simulink model "KF"  (R2025b)
settings: Solver=VariableStepAuto  StartTime=0.0  StopTime=35  RelTol=1e-3
StopFcn:
  | % -----------------------------
  | %   Kalman Filter Visualization
  | % -----------------------------
  | 
  | % 안전하게 데이터 존재 여부 확인
  | if evalin('base','exist(''out'',''var'')')
  | 
  |     % out 구조체 불러오기
  |     data = evalin('base','out');
  | 
  |     % Timeseries 는 .Time, .Data 로 접근
  |     t = data.z_out.Time;
  | 
  |     % 관측 z_k = [x, y]
  |     z_x = data.z_out.Data(:,1);
  |     z_y = data.z_out.Data(:,2);
  | 
  |     % x_pred = [x vx y vy]
  |     xpred_x = data.x_pred.Data(:,1);
  |     xpred_y = data.x_pred.Data(:,3);
  | 
  |     % x_est = [x vx y vy]
  |     xest_x = data.x_est.Data(:,1);
  |     xest_y = data.x_est.Data(:,3);
  | 
  |     figure; hold on; grid on;
  | 
  |     % ---- X plot ----
  |     subplot(2,1,1); hold on; grid on;
  |     plot(t, z_x,'ro','DisplayName','Observed X');
  |     plot(t, xpred_x,'b--','LineWidth',1.3,'DisplayName','Predicted X');
  |     plot(t, xest_x,'g-','LineWidth',1.3,'DisplayName','Estimated X');
  |     xlabel('Time'); ylabel('X'); title('X Position');
  |     legend;
  | 
  |     % ---- Y plot ----
  |     subplot(2,1,2); hold on; grid on;
  |     plot(t, z_y,'ro','DisplayName','Observed Y');
  |     plot(t, xpred_y,'b--','LineWidth',1.3,'DisplayName','Predicted Y');
  |     plot(t, xest_y,'g-','LineWidth',1.3,'DisplayName','Estimated Y');
  |     xlabel('Time'); ylabel('Y'); title('Y Position');
  |     legend;
  | 
  | else
  |     disp('ERROR: out 구조체가 workspace에 없습니다.');
  | end
libraries: simulink x2, matrix_library x2
settings Model: Creator=xox  LastModifiedBy=xox
settings OptimizationCC: BlockReduction=off  DefaultParameterBehavior=Inlined  BufferReuse=off

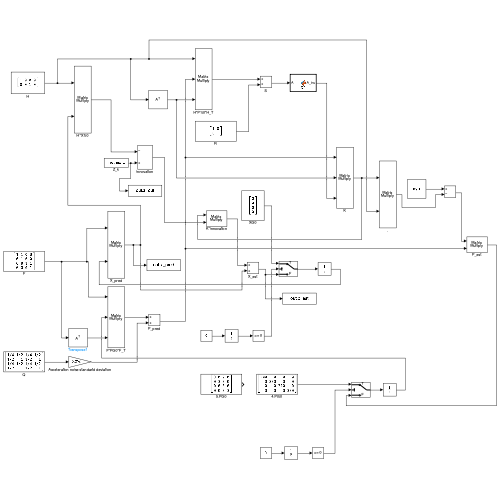
[thumbnail: Simulink's stored preview of the top-level diagram]
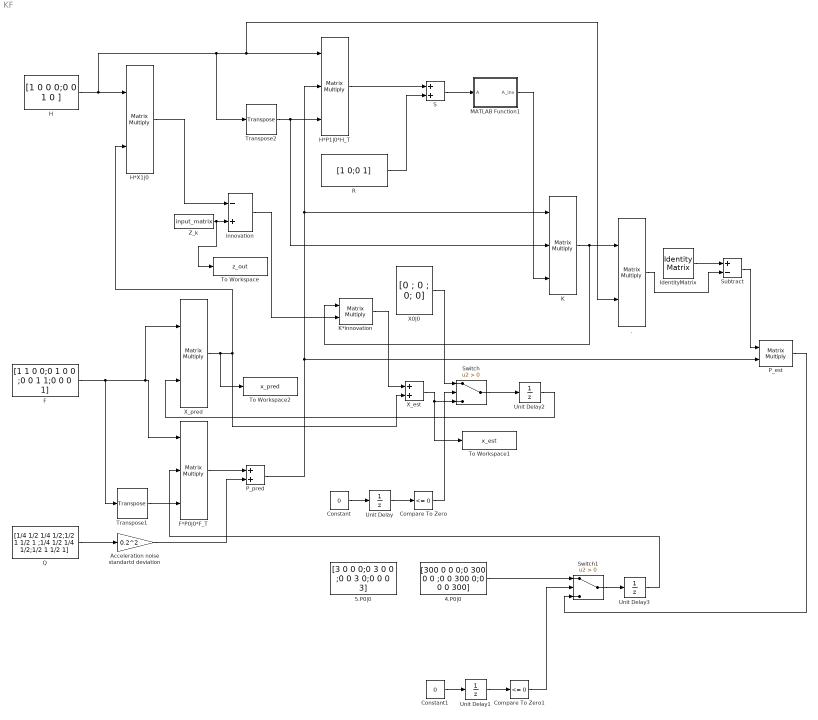
== system KF ==
  . : Product  Multiplication=Matrix(*)
  4.P0|0 : Constant  Value=[300 0 0 0;0 300 0 0 ;0 0 300 0;0 0 0 300]  VectorParams1D=off
  5.P0|0 : Constant  Value=[3 0 0 0;0 3 0 0 ;0 0 3 0;0 0 0 3]  VectorParams1D=off
  Acceleration noise standartd deviation : Gain  Gain=0.2^2
  Compare To Zero : simulink/Logic and Bit Operations/Compare To Zero  relop=<=  OutDataTypeStr=boolean
  Compare To Zero1 : simulink/Logic and Bit Operations/Compare To Zero  relop=<=  OutDataTypeStr=boolean
  Constant : Constant  Value=0
  Constant1 : Constant  Value=0
  F : Constant  Value=[1 1 0 0;0 1 0 0 ;0 0 1 1;0 0 0 1]  VectorParams1D=off
  F*P0|0*F_T : Product  Inputs=3  Multiplication=Matrix(*)
  H : Constant  Value=[1 0 0 0;0 0 1 0 ]  VectorParams1D=off
  H*P1|0*H_T : Product  Inputs=3  Multiplication=Matrix(*)
  H*X1|0 : Product  Multiplication=Matrix(*)
  IdentityMatrix : IdentityMatrix  OutputDimensions=4
  K : Product  Inputs=3  Multiplication=Matrix(*)
  K*innovation : Product  Multiplication=Matrix(*)
  MATLAB Function1 : MATLAB Function  TreatAsAtomicUnit=on
  P_est : Product  Multiplication=Matrix(*)
  P_pred : Sum
  Q : Constant  Value=[1/4 1/2 1/4 1/2;1/2 1 1/2 1 ;1/4 1/2 1/4 1/2;1/2 1 1/2 1]  VectorParams1D=off
  R : Constant  Value=[1 0;0 1]  VectorParams1D=off
  S : Sum
  Subtract : Sum  Inputs=+-
  Switch : Switch  Criteria=u2 > Threshold  SaturateOnIntegerOverflow=off  InputSameDT=off
  Switch1 : Switch  Criteria=u2 > Threshold  SaturateOnIntegerOverflow=off  InputSameDT=off
  To Workspace : ToWorkspace  VariableName=z_out  SaveFormat=Timeseries  SampleTime=-1
  To Workspace1 : ToWorkspace  VariableName=x_est  SaveFormat=Timeseries  SampleTime=-1
  To Workspace2 : ToWorkspace  VariableName=x_pred  SaveFormat=Timeseries  SampleTime=-1
  Transpose1 : matrix_library/Transpose
  Transpose2 : matrix_library/Transpose
  Unit Delay{,1..3} (4 alike) : UnitDelay  SampleTime=-1  HasFrameUpgradeWarning=on
  X0|0 : Constant  Value=[0 ; 0 ; 0; 0]  VectorParams1D=off
  X_est : Sum
  X_pred : Product  Multiplication=Matrix(*)
  Z_k : FromWorkspace  VariableName=input_matrix  SampleTime=-1
  innovation : Sum  Inputs=-+
  wires:
  F/1 -> Transpose1/1, X_pred/1, F*P0|0*F_T/1
  Transpose1/1 -> F*P0|0*F_T/3
  Q/1 -> Acceleration noise standartd deviation/1
  F*P0|0*F_T/1 -> P_pred/1
  Acceleration noise standartd deviation/1 -> P_pred/2
  H*X1|0/1 -> innovation/1
  P_pred/1 -> P_est/2, K/1, H*P1|0*H_T/2
  H/1 -> Transpose2/1, ./2, H*P1|0*H_T/1, H*X1|0/1
  R/1 -> S/2
  H*P1|0*H_T/1 -> S/1
  Transpose2/1 -> K/2, H*P1|0*H_T/3
  S/1 -> MATLAB Function1/1(A)
  MATLAB Function1/1(A_inv) -> K/3
  IdentityMatrix/1 -> Subtract/1
  K/1 -> K*innovation/1, ./1
  ./1 -> Subtract/2
  Subtract/1 -> P_est/1
  X_pred/1 -> To Workspace2/1, X_est/2, H*X1|0/2
  Z_k/1 -> To Workspace/1, innovation/2
  innovation/1 -> K*innovation/2
  K*innovation/1 -> X_est/1
  Constant/1 -> Unit Delay/1
  Unit Delay/1 -> Compare To Zero/1
  Compare To Zero/1 -> Switch/2
  X_est/1 -> Switch/3, To Workspace1/1
  X0|0/1 -> Switch/1
  P_est/1 -> Switch1/3
  Unit Delay1/1 -> Compare To Zero1/1
  Constant1/1 -> Unit Delay1/1
  Compare To Zero1/1 -> Switch1/2
  4.P0|0/1 -> Switch1/1
  Switch/1 -> Unit Delay2/1
  Unit Delay2/1 -> X_pred/2
  Switch1/1 -> Unit Delay3/1
  Unit Delay3/1 -> F*P0|0*F_T/2

== matlab function KF/MATLAB Function1 ==
  data: A input; A_inv output
function A_inv = fcn(A)
A_inv = inv(A);
